simulink model "chap5_3sim"  (Simulink 5.1)
settings: Solver=ode45  StartTime=0.0  StopTime=30  RelTol=1e-3
settings Model: LastModifiedBy=liu  ExtModeTrigMode=oneshot  ExtModeArmWhenConnect=off  LimitDataPoints=off  ProdHWDeviceType=Microprocessor

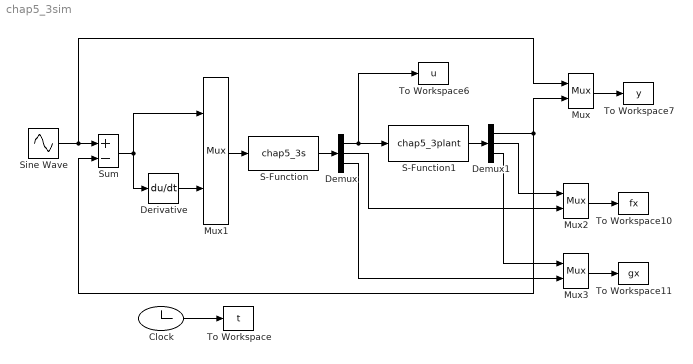
== system chap5_3sim ==
  Clock : Clock
  Demux : Demux  Outputs=3
  Demux1 : Demux  Outputs=3
  Derivative : Derivative
  Mux{,1..3} (4 alike) : Mux  Inputs=2
  S-Function : S-Function  FunctionName=chap5_3s
  S-Function1 : S-Function  FunctionName=chap5_3plant
  Sine Wave : Sin  Amplitude=0.1  SampleTime=0
  Sum : Sum  Inputs=+-  SaturateOnIntegerOverflow=on  InputSameDT=on
  To Workspace : ToWorkspace  VariableName=t  SampleTime=-1  SaveFormat=Array
  To Workspace10 : ToWorkspace  VariableName=fx  SampleTime=-1  SaveFormat=Array
  To Workspace11 : ToWorkspace  VariableName=gx  SampleTime=-1  SaveFormat=Array
  To Workspace6 : ToWorkspace  VariableName=u  SampleTime=-1  SaveFormat=Array
  To Workspace7 : ToWorkspace  VariableName=y  SampleTime=-1  SaveFormat=Array
  wires:
  Mux1/1 -> S-Function/1
  S-Function/1 -> Demux/1
  Sum/1 -> Mux1/1, Derivative/1
  Sine Wave/1 -> Sum/1, Mux/1
  Derivative/1 -> Mux1/2
  Demux/1 -> S-Function1/1, To Workspace6/1
  S-Function1/1 -> Demux1/1
  Clock/1 -> To Workspace/1
  Mux/1 -> To Workspace7/1
  Demux1/1 -> Sum/2, Mux/2
  Demux1/2 -> Mux2/1
  Mux2/1 -> To Workspace10/1
  Demux/2 -> Mux2/2
  Demux1/3 -> Mux3/1
  Mux3/1 -> To Workspace11/1
  Demux/3 -> Mux3/2
